simulink model "q2d"  (R2017a)
settings: Solver=VariableStepAuto  StartTime=0.0  StopTime=10.0  RelTol=1e-3
settings Model: Creator=adamhzp  LastModifiedBy=adamhzp

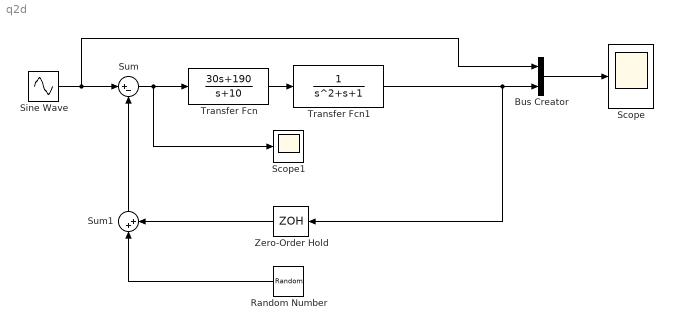
== system q2d ==
  Bus Creator : BusCreator  Inputs=2
  Random Number : RandomNumber  Variance=0.01  SampleTime=0.005
  Scope : Scope
  Scope1 : Scope
  Sine Wave : Sin  SampleTime=0
  Sum : Sum  Inputs=|+-
  Sum1 : Sum  Inputs=|++
  Transfer Fcn : TransferFcn  Numerator=[30 190]  Denominator=[1 10]
  Transfer Fcn1 : TransferFcn  Denominator=[1 1 1]
  Zero-Order Hold : ZeroOrderHold  SampleTime=0.005
  wires:
  Transfer Fcn/1 -> Transfer Fcn1/1
  Sine Wave/1 -> Bus Creator/1, Sum/1
  Bus Creator/1 -> Scope/1
  Sum/1 -> Scope1/1, Transfer Fcn/1
  Transfer Fcn1/1 -> Zero-Order Hold/1, Bus Creator/2
  Random Number/1 -> Sum1/1
  Zero-Order Hold/1 -> Sum1/2
  Sum1/1 -> Sum/2
